simulink model "proyecto"  (R2021a)
settings: Solver=VariableStepAuto  StartTime=0.0  StopTime=10.0  RelTol=1e-3
model workspace (MAT data in the model file):
  Cts = Simulink.Parameter
  Cts.DataType = 'auto'
  Cts.Dimensions = [0 0]
  J_eq = Simulink.Parameter
  J_eq.DataType = 'auto'
  J_eq.Dimensions = [0 0]
  Jeq = Simulink.Parameter
  Jeq.DataType = 'auto'
  Jeq.Dimensions = [0 0]
  Ke = Simulink.Parameter
  Ke.DataType = 'auto'
  Ke.Dimensions = [0 0]
  Ksa = Simulink.Parameter
  Ksa.DataType = 'auto'
  Ksa.Dimensions = [0 0]
  Ksia = Simulink.Parameter
  Ksia.DataType = 'auto'
  Ksia.Dimensions = [0 0]
  Kt = Simulink.Parameter
  Kt.DataType = 'auto'
  Kt.Dimensions = [0 0]
  Ktheta = Simulink.Parameter
  Ktheta.DataType = 'auto'
  Ktheta.Dimensions = [0 0]
  Kw = Simulink.Parameter
  Kw.DataType = 'auto'
  Kw.Dimensions = [0 0]
  Ld = Simulink.Parameter
  Ld.DataType = 'auto'
  Ld.Dimensions = [0 0]
  LdP = Simulink.Parameter
  LdP.DataType = 'auto'
  LdP.Dimensions = [0 0]
  Lls = Simulink.Parameter
  Lls.DataType = 'auto'
  Lls.Dimensions = [0 0]
  Lq = Simulink.Parameter
  Lq.DataType = 'auto'
  Lq.Dimensions = [0 0]
  LqP = Simulink.Parameter
  LqP.DataType = 'auto'
  LqP.Dimensions = [0 0]
  Pp = Simulink.Parameter
  Pp.DataType = 'auto'
  Pp.Dimensions = [0 0]
  R0 = Simulink.Parameter
  R0.DataType = 'auto'
  R0.Dimensions = [0 0]
  R0P = Simulink.Parameter
  R0P.DataType = 'auto'
  R0P.Dimensions = [0 0]
  Rd = Simulink.Parameter
  Rd.DataType = 'auto'
  Rd.Dimensions = [0 0]
  RdP = Simulink.Parameter
  RdP.DataType = 'auto'
  RdP.Dimensions = [0 0]
  Rq = Simulink.Parameter
  Rq.DataType = 'auto'
  Rq.Dimensions = [0 0]
  RqP = Simulink.Parameter
  RqP.DataType = 'auto'
  RqP.Dimensions = [0 0]
  Rs = Simulink.Parameter
  Rs.DataType = 'auto'
  Rs.Dimensions = [0 0]
  RsP = Simulink.Parameter
  RsP.DataType = 'auto'
  RsP.Dimensions = [0 0]
  Rs_ref = Simulink.Parameter
  Rs_ref.DataType = 'auto'
  Rs_ref.Dimensions = [0 0]
  Rtsamb = Simulink.Parameter
  Rtsamb.DataType = 'auto'
  Rtsamb.Dimensions = [0 0]
  T_amb = Simulink.Parameter
  T_amb.DataType = 'auto'
  T_amb.Dimensions = [0 0]
  Ts_ref = Simulink.Parameter
  Ts_ref.DataType = 'auto'
  Ts_ref.Dimensions = [0 0]
  a_cu = Simulink.Parameter
  a_cu.DataType = 'auto'
  a_cu.Dimensions = [0 0]
  b_eq = Simulink.Parameter
  b_eq.DataType = 'auto'
  b_eq.Dimensions = [0 0]
  ba = Simulink.Parameter
  ba.DataType = 'auto'
  ba.Dimensions = [0 0]
  beqP = Simulink.Parameter
  beqP.DataType = 'auto'
  beqP.Dimensions = [0 0]
  lambda_m = Simulink.Parameter
  lambda_m.DataType = 'auto'
  lambda_m.Dimensions = [0 0]
  r = Simulink.Parameter
  r.DataType = 'auto'
  r.Dimensions = [0 0]
values from neighbouring files (symbols this model uses):
  a_cu = 3.9e-3    (= 0.0039)    [Datos.m]
  b_eq = 15.000e-6    (= 1.5e-05)    [Datos.m]
  ba = 0.0113    [Datos.m]
  Cts = 0.818    [Datos.m]
  Id_0 = 0    [Datos.m]
  J_eq = 5.6509e-6    (= 5.6509e-06)    [Datos.m]
  Ksa = 9.0414    [Datos.m]
  Ksia = 2893.2608    [Datos.m]
  Ktheta = 6397.34    [Datos.m]
  Kw = 10.2234e6    (= 10223400)    [Datos.m]
  lambda_m = 0.01546    [Datos.m]
  Ld = 6.6e-3    (= 0.0066)    [Datos.m]
  Lls = 0.8e-3    (= 0.0008)    [Datos.m]
  Lq = 5.8e-3    (= 0.0058)    [Datos.m]
  Pp = 3.01    [Datos.m]
  r = 314.3008    [Datos.m]
  Rs = 1.02    [Datos.m]
  Rs_ref = 1.02    [Datos.m]
  Rtsamb = 146.7    [Datos.m]
  T_0 = 40.0    (= 40)    [Datos.m]
  T_amb = 40    [Datos.m]
  Ts_ref = 40    [Datos.m]
undefined symbols (not defined in the file or in its folder): sigbuilder_block
(part 1 of 3)
settings Model: Creator=jpss8  LastModifiedBy=jpss8

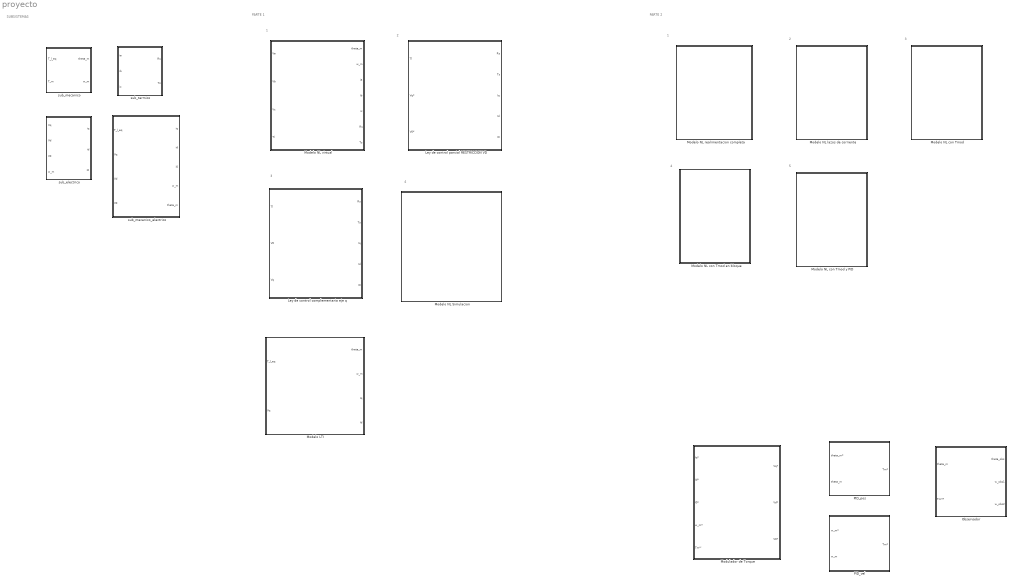
== system proyecto ==
  note: 1
  note: PARTE 2
  note: PARTE 1
  note: SUBSISTEMAS
  note: 2
  note: 3
  note: 4
  note: 5
  note: 1
  note: 2
  note: 3
  note: 4
  Ley de control complementaria eje q : Subsystem
  Ley de control parcial RESTRICCION VD : Subsystem
  Modelo LTI : Subsystem
  Modelo NL Simulacion : Subsystem
  Modelo NL con Tmod : Subsystem
  Modelo NL con Tmod en bloque : Subsystem
  Modelo NL con Tmod y PID : Subsystem
  Modelo NL lazos de corriente : Subsystem
  Modelo NL realimentacion completa : Subsystem
  Modelo NL virtual : Subsystem
  Modulador de Torque : Subsystem
  Observador : Subsystem
  PID_pos : Subsystem
  PID_vel : Subsystem
  sub_electrico : Subsystem
  sub_mecanico : Subsystem
  sub_mecanico_electrico : Subsystem
  sub_termico : Subsystem

== system proyecto/Ley de control complementaria eje q ==
  note: CONTROLADOR (Ley complementaria eje q)
  note: SISTEMA FÍSICO
  Tl : Inport
  V0 : Inport  Port=2
  Vq : Inport  Port=3
  Constant : Constant  Value=lambda_m
  Gain : Gain  Gain=Pp
  Gain1 : Gain  Gain=1/r
  Gain2 : Gain  Gain=Pp
  Gain3 : Gain  Gain=-Lq
  Gain4 : Gain  Gain=Ld
  Gain8 : Gain  Gain=Pp
  Modulador de Tensión : Subsystem
  Product : Product
  Product1 : Product
  Sensor de Corriente : Subsystem
  Sensor de posición : Gain
  Sensor de velocidad : Gain
  Sum : Sum  Inputs=|++
  Sum1 : Sum  Inputs=|++
  inverse_park_transform : MATLAB Function  TreatAsAtomicUnit=on
  inverse_park_transform1 : MATLAB Function  TreatAsAtomicUnit=on
  park_transform : MATLAB Function  TreatAsAtomicUnit=on
  park_transform1 : MATLAB Function  TreatAsAtomicUnit=on
  sub_mecanico_electrico : Subsystem
  sub_termico : Subsystem
  Rs : Outport
  Ts : Outport  Port=2
  Iq : Outport  Port=3
  Id : Outport  Port=4
  I0 : Outport  Port=5
  wires:
  Gain/1 -> inverse_park_transform/4(theta_r), park_transform/4(theta_r)
  Tl/1 -> Gain1/1
  Gain1/1 -> sub_mecanico_electrico/4(V0)
  sub_mecanico_electrico/1(iq) -> inverse_park_transform/1(fq)
  park_transform/1(fq) -> sub_mecanico_electrico/1(T_l_eq)
  park_transform/2(fd) -> sub_mecanico_electrico/2(Vq)
  sub_mecanico_electrico/2(id) -> inverse_park_transform/2(fd)
  sub_mecanico_electrico/3(i0) -> inverse_park_transform/3(f0)
  sub_mecanico_electrico/5(theta_m) -> Sensor de posición/1, Gain/1
  sub_termico/1(Rs) -> Rs/1
  sub_termico/2(Ts) -> Ts/1
  sub_mecanico_electrico/4(w_m) -> Sensor de velocidad/1
  park_transform/3(f0) -> sub_mecanico_electrico/3(Vd)
  Gain8/1 -> park_transform1/4(theta_r), inverse_park_transform1/4(theta_r)  "theta_r*"
  Modulador de Tensión/1(Out1) -> park_transform/1(fa)  "Va"
  Modulador de Tensión/2(Out2) -> park_transform/2(fb)  "Vb"
  Modulador de Tensión/3(Out3) -> park_transform/3(fc)  "Vc"
  Sensor de Corriente/1(Out1) -> park_transform1/1(fa), sub_termico/1(ia)
  Sensor de Corriente/3(Out3) -> park_transform1/3(fc), sub_termico/3(ic)
  Sensor de Corriente/2(Out2) -> sub_termico/2(ib), park_transform1/2(fb)
  inverse_park_transform/1(fa) -> Sensor de Corriente/1(In1)
  inverse_park_transform/2(fb) -> Sensor de Corriente/2(In2)
  inverse_park_transform/3(fc) -> Sensor de Corriente/3(In3)
  park_transform1/1(fq) -> Gain3/1, Iq/1  "Iq*"
  park_transform1/2(fd) -> Gain4/1, Id/1  "Id*"
  park_transform1/3(f0) -> I0/1  "I0*"
  Product/1 -> inverse_park_transform1/2(fd)  "Vd*"
  V0/1 -> inverse_park_transform1/3(f0)
  inverse_park_transform1/2(fb) -> Modulador de Tensión/2(fb)  "Vb*"
  inverse_park_transform1/3(fc) -> Modulador de Tensión/3(fc)  "Vc*"
  inverse_park_transform1/1(fa) -> Modulador de Tensión/1(fa)  "Va*"
  Sensor de posición/1 -> Gain8/1  "theta_m*"
  Sensor de velocidad/1 -> Gain2/1  "w_m*"
  Gain2/1 -> Product1/1, Product/1
  Gain3/1 -> Product/2
  Gain4/1 -> Sum/1
  Sum/1 -> Product1/2  "lambda_m + Ld*Id"
  Constant/1 -> Sum/2
  Product1/1 -> Sum1/2
  Sum1/1 -> inverse_park_transform1/1(fq)  "Vq*"
  Vq/1 -> Sum1/1

== system proyecto/Ley de control parcial RESTRICCION VD ==
  note: CONTROLADOR (Restricción Vd)
  note: SISTEMA FÍSICO
  Tl : Inport
  Vq* : Inport  Port=2
  V0* : Inport  Port=3
  Gain : Gain  Gain=Pp
  Gain1 : Gain  Gain=1/r
  Gain2 : Gain  Gain=Pp
  Gain3 : Gain  Gain=-Lq
  Gain8 : Gain  Gain=Pp
  Modulador de Tensión : Subsystem
  Product : Product
  Sensor de Corriente : Subsystem
  Sensor de posición : Gain
  Sensor de velocidad : Gain
  inverse_park_transform : MATLAB Function  TreatAsAtomicUnit=on
  inverse_park_transform1 : MATLAB Function  TreatAsAtomicUnit=on
  park_transform : MATLAB Function  TreatAsAtomicUnit=on
  park_transform1 : MATLAB Function  TreatAsAtomicUnit=on
  sub_mecanico_electrico : Subsystem
  sub_termico : Subsystem
  Rs : Outport
  Ts : Outport  Port=2
  Iq : Outport  Port=3
  Id : Outport  Port=4
  I0 : Outport  Port=5
  wires:
  Gain/1 -> inverse_park_transform/4(theta_r), park_transform/4(theta_r)
  Tl/1 -> Gain1/1
  Gain1/1 -> sub_mecanico_electrico/4(V0)
  sub_mecanico_electrico/1(iq) -> inverse_park_transform/1(fq)
  park_transform/1(fq) -> sub_mecanico_electrico/1(T_l_eq)
  park_transform/2(fd) -> sub_mecanico_electrico/2(Vq)
  sub_mecanico_electrico/2(id) -> inverse_park_transform/2(fd)
  sub_mecanico_electrico/3(i0) -> inverse_park_transform/3(f0)
  sub_mecanico_electrico/5(theta_m) -> Sensor de posición/1, Gain/1
  sub_termico/1(Rs) -> Rs/1
  sub_termico/2(Ts) -> Ts/1
  sub_mecanico_electrico/4(w_m) -> Sensor de velocidad/1
  park_transform/3(f0) -> sub_mecanico_electrico/3(Vd)
  Gain8/1 -> park_transform1/4(theta_r), inverse_park_transform1/4(theta_r)  "theta_r*"
  Modulador de Tensión/1(Out1) -> park_transform/1(fa)  "Va"
  Modulador de Tensión/2(Out2) -> park_transform/2(fb)  "Vb"
  Modulador de Tensión/3(Out3) -> park_transform/3(fc)  "Vc"
  Sensor de Corriente/1(Out1) -> park_transform1/1(fa), sub_termico/1(ia)
  Sensor de Corriente/3(Out3) -> sub_termico/3(ic), park_transform1/3(fc)
  Sensor de Corriente/2(Out2) -> sub_termico/2(ib), park_transform1/2(fb)
  inverse_park_transform/1(fa) -> Sensor de Corriente/1(In1)
  inverse_park_transform/2(fb) -> Sensor de Corriente/2(In2)
  inverse_park_transform/3(fc) -> Sensor de Corriente/3(In3)
  park_transform1/1(fq) -> Gain3/1, Iq/1  "Iq*"
  park_transform1/2(fd) -> Id/1
  park_transform1/3(f0) -> I0/1
  Vq*/1 -> inverse_park_transform1/1(fq)
  Product/1 -> inverse_park_transform1/2(fd)  "Vd*"
  V0*/1 -> inverse_park_transform1/3(f0)
  inverse_park_transform1/2(fb) -> Modulador de Tensión/2(fb)  "Vb*"
  inverse_park_transform1/3(fc) -> Modulador de Tensión/3(fc)  "Vc*"
  inverse_park_transform1/1(fa) -> Modulador de Tensión/1(fa)  "Va*"
  Sensor de posición/1 -> Gain8/1  "theta_m*"
  Sensor de velocidad/1 -> Gain2/1  "w_m*"
  Gain2/1 -> Product/1
  Gain3/1 -> Product/2

== system proyecto/Modelo LTI ==
  T_l_eq : Inport
  Vq : Inport  Port=2
  Constant1 : Constant  Value=0
  Gain : Gain  Gain=3/2*Pp*lambda_m
  Gain1 : Gain  Gain=Pp*lambda_m
  Gain12 : Gain  Gain=Rs
  Gain13 : Gain  Gain=1/Ld
  Gain2 : Gain  Gain=Rs
  Gain3 : Gain  Gain=1/Lq
  Gain4 : Gain  Gain=1/J_eq
  Gain5 : Gain  Gain=b_eq
  Integrator{,1..3} (4 alike) : Integrator
  Sum : Sum  Inputs=-+-
  Sum1 : Sum  Inputs=+--
  Sum5 : Sum  Inputs=|+-
  theta_m : Outport
  w_m : Outport  Port=2
  Iq : Outport  Port=3
  Id : Outport  Port=4
  wires:
  Integrator1/1 -> theta_m/1
  Gain4/1 -> Integrator/1
  T_l_eq/1 -> Sum/1
  Sum/1 -> Gain4/1
  Integrator/1 -> Integrator1/1, Gain1/1, Gain5/1, w_m/1
  Gain5/1 -> Sum/3
  Gain/1 -> Sum/2
  Vq/1 -> Sum1/1
  Gain1/1 -> Sum1/2
  Gain2/1 -> Sum1/3
  Sum1/1 -> Gain3/1
  Gain3/1 -> Integrator2/1
  Integrator2/1 -> Iq/1, Gain2/1, Gain/1  "Iq"
  Integrator3/1 -> Id/1, Gain12/1  "Id"
  Sum5/1 -> Gain13/1
  Gain13/1 -> Integrator3/1
  Constant1/1 -> Sum5/1
  Gain12/1 -> Sum5/2

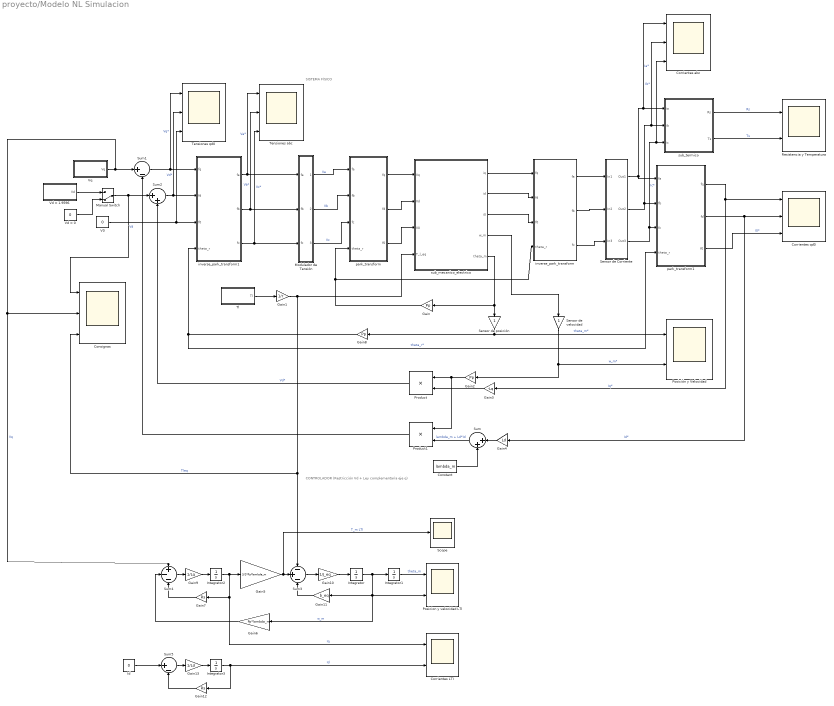
== system proyecto/Modelo NL Simulacion ==
  note: SISTEMA FÍSICO
  note: CONTROLADOR (Restricción Vd + Ley complementaria eje q)
  Consignas : Scope  NumInputPorts=3
  Constant : Constant  Value=lambda_m
  Corrientes LTI : Scope  NumInputPorts=2
  Corrientes abc : Scope  NumInputPorts=3
  Corrientes qd0 : Scope  NumInputPorts=3
  Gain : Gain  Gain=Pp
  Gain1 : Gain  Gain=1/r
  Gain10 : Gain  Gain=1/J_eq
  Gain11 : Gain  Gain=b_eq
  Gain12 : Gain  Gain=Rs
  Gain13 : Gain  Gain=1/Ld
  Gain2 : Gain  Gain=Pp
  Gain3 : Gain  Gain=-Lq
  Gain4 : Gain  Gain=Ld
  Gain5 : Gain  Gain=3/2*Pp*lambda_m
  Gain6 : Gain  Gain=Pp*lambda_m
  Gain7 : Gain  Gain=Rs
  Gain8 : Gain  Gain=Pp
  Gain9 : Gain  Gain=1/Lq
  Id : Constant  Value=0
  Integrator : Integrator
  Integrator1 : Integrator
  Integrator2 : Integrator
  Integrator3 : Integrator  InitialCondition=Id_0
  Manual Switch : ManualSwitch  CurrentSetting=0
  Modulador de Tensión : Subsystem
  Posicion y velocidad LTI : Scope  NumInputPorts=2
  Posición y Velocidad : Scope  NumInputPorts=2
  Product : Product
  Product1 : Product
  Resistencia y Temperatura : Scope  NumInputPorts=2
  Scope : Scope
  Sensor de Corriente : Subsystem
  Sensor de posición : Gain
  Sensor de velocidad : Gain
  Sum : Sum  Inputs=|++
  Sum1 : Sum  Inputs=|+-
  Sum2 : Sum  Inputs=|++
  Sum3 : Sum  Inputs=-+-
  Sum4 : Sum  Inputs=+--
  Sum5 : Sum  Inputs=|+-
  Tensiones abc : Scope  NumInputPorts=3
  Tensiones qd0 : Scope  NumInputPorts=3
  Tl : Subsystem  Tag=STV Subsys  LoadFcn=sigbuilder_block('load');  StartFcn=sigbuilder_block('start');  StopFcn=sigbuilder_block('stop');  ClipboardFcn=sigbuilder_block('clipboard');  mask(Sigbuilder block){tuvar=[0:10]}
      mask help: Simulink:masks:SigbuilderBlock_MD
      mask init:
      | if ~strcmp(get_param(bdroot(gcbh),'SimulationStatus'),'stopped') tuvar = sigbuilder_block('maskInit'); end
      settings: CopyFcn=sigbuilder_block('copy');  DeleteFcn=sigbuilder_block('delete');  ModelCloseFcn=sigbuilder_block('modelClose');  PreSaveFcn=sigbuilder_block('preSave');  PauseFcn=sigbuilder_block('pause');  ContinueFcn=sigbuilder_block('continue');  NameChangeFcn=sigbuilder_block('namechange');  OpenFcn=sigbuilder_block('open',[5.5 30 1269 678 ]);  CloseFcn=sigbuilder_block('close');
      mask Display: plot(0, 0, 100, 100,[2, 2, 32, 32, 2], [68, 8, 8, 68, 68],[32, 2], [38, 38], [32, 19, 2],[53, 60, 44], [32, 17, 17, 2],[16, 16, 31, 31]);txt = getActiveGroup(gcbh);text(2, 100, txt,'verticalAlignment', 'top');
  V0 : Constant  Value=0
  Vd = 0 : Constant  Value=0
  Vd = 1.9596 : Subsystem  Tag=STV Subsys  LoadFcn=sigbuilder_block('load');  StartFcn=sigbuilder_block('start');  StopFcn=sigbuilder_block('stop');  ClipboardFcn=sigbuilder_block('clipboard');  mask(Sigbuilder block){tuvar=[0:10]}
      mask help: Simulink:masks:SigbuilderBlock_MD
      mask init:
      | if ~strcmp(get_param(bdroot(gcbh),'SimulationStatus'),'stopped') tuvar = sigbuilder_block('maskInit'); end
      settings: CopyFcn=sigbuilder_block('copy');  DeleteFcn=sigbuilder_block('delete');  ModelCloseFcn=sigbuilder_block('modelClose');  PreSaveFcn=sigbuilder_block('preSave');  PauseFcn=sigbuilder_block('pause');  ContinueFcn=sigbuilder_block('continue');  NameChangeFcn=sigbuilder_block('namechange');  OpenFcn=sigbuilder_block('open',[5.5 30 1269 678 ]);  CloseFcn=sigbuilder_block('close');
      mask Display: plot(0, 0, 100, 100,[2, 2, 32, 32, 2], [68, 8, 8, 68, 68],[32, 2], [38, 38], [32, 19, 2],[53, 60, 44], [32, 17, 17, 2],[16, 16, 31, 31]);txt = getActiveGroup(gcbh);text(2, 100, txt,'verticalAlignment', 'top');
  Vq : Subsystem  Tag=STV Subsys  LoadFcn=sigbuilder_block('load');  StartFcn=sigbuilder_block('start');  StopFcn=sigbuilder_block('stop');  ClipboardFcn=sigbuilder_block('clipboard');  mask(Sigbuilder block){tuvar=[0:10]}
      mask help: Simulink:masks:SigbuilderBlock_MD
      mask init:
      | if ~strcmp(get_param(bdroot(gcbh),'SimulationStatus'),'stopped') tuvar = sigbuilder_block('maskInit'); end
      settings: CopyFcn=sigbuilder_block('copy');  DeleteFcn=sigbuilder_block('delete');  ModelCloseFcn=sigbuilder_block('modelClose');  PreSaveFcn=sigbuilder_block('preSave');  PauseFcn=sigbuilder_block('pause');  ContinueFcn=sigbuilder_block('continue');  NameChangeFcn=sigbuilder_block('namechange');  OpenFcn=sigbuilder_block('open',[5.5 30 1269 678 ]);  CloseFcn=sigbuilder_block('close');
      mask Display: plot(0, 0, 100, 100,[2, 2, 32, 32, 2], [68, 8, 8, 68, 68],[32, 2], [38, 38], [32, 19, 2],[53, 60, 44], [32, 17, 17, 2],[16, 16, 31, 31]);txt = getActiveGroup(gcbh);text(2, 100, txt,'verticalAlignment', 'top');
  inverse_park_transform : MATLAB Function  TreatAsAtomicUnit=on
  inverse_park_transform1 : MATLAB Function  TreatAsAtomicUnit=on
  park_transform : MATLAB Function  TreatAsAtomicUnit=on
  park_transform1 : MATLAB Function  TreatAsAtomicUnit=on
  sub_mecanico_electrico : Subsystem
  sub_termico : Subsystem
  wires:
  park_transform1/3(f0) -> Corrientes qd0/3  "I0*"
  Product1/1 -> Sum1/2
  inverse_park_transform/2(fb) -> Sensor de Corriente/2(In2)
  Integrator1/1 -> Posicion y velocidad LTI/1  "theta_m"
  sub_termico/1(Rs) -> Resistencia y Temperatura/1  "Rs"
  Gain6/1 -> Sum4/2
  Gain5/1 -> Scope/1, Sum3/2  "T_m LTI"
  Sensor de Corriente/1(Out1) -> park_transform1/1(fa), Corrientes abc/1, sub_termico/1(ia)  "Ia*"
  Gain13/1 -> Integrator3/1
  sub_mecanico_electrico/1(iq) -> inverse_park_transform/1(fq)
  Gain7/1 -> Sum4/3
  Modulador de Tensión/1(Out1) -> park_transform/1(fa)  "Va"
  park_transform/1(fq) -> sub_mecanico_electrico/1(Vq)
  Id/1 -> Sum5/1
  Sum5/1 -> Gain13/1
  Gain12/1 -> Sum5/2
  park_transform1/1(fq) -> Gain3/1, Corrientes qd0/1  "Iq*"
  Sum2/1 -> Tensiones qd0/2, inverse_park_transform1/2(fd)  "Vd*"
  Gain9/1 -> Integrator2/1
  Gain11/1 -> Sum3/3
  park_transform1/2(fd) -> Gain4/1, Corrientes qd0/2  "Id*"
  Gain10/1 -> Integrator/1
  Sum4/1 -> Gain9/1
  Gain8/1 -> park_transform1/4(theta_r), inverse_park_transform1/4(theta_r)  "theta_r*"
  Sum3/1 -> Gain10/1
  Integrator2/1 -> Gain7/1, Corrientes LTI/1, Gain5/1  "Iq"
  Integrator/1 -> Gain6/1, Posicion y velocidad LTI/2, Gain11/1, Integrator1/1  "w_m"
  Vd = 0/1 -> Manual Switch/2
  Modulador de Tensión/3(Out3) -> park_transform/3(fc)  "Vc"
  park_transform/3(f0) -> sub_mecanico_electrico/3(V0)
  Sensor de velocidad/1 -> Gain2/1, Posición y Velocidad/2  "w_m*"
  Vd = 1.9596/1(Vd) -> Manual Switch/1
  park_transform/2(fd) -> sub_mecanico_electrico/2(Vd)
  Sensor de Corriente/2(Out2) -> park_transform1/2(fb), Corrientes abc/2, sub_termico/2(ib)  "Ib*"
  inverse_park_transform/3(fc) -> Sensor de Corriente/3(In3)
  Manual Switch/1 -> Consignas/1, Sum2/1  "Vd"
  Sensor de Corriente/3(Out3) -> park_transform1/3(fc), Corrientes abc/3, sub_termico/3(ic)  "Ic*"
  inverse_park_transform1/1(fa) -> Tensiones abc/1, Modulador de Tensión/1(fa)  "Va*"
  Tl/1(Tl) -> Gain1/1
  sub_mecanico_electrico/4(w_m) -> Sensor de velocidad/1
  Gain3/1 -> Product/2
  inverse_park_transform/1(fa) -> Sensor de Corriente/1(In1)
  Modulador de Tensión/2(Out2) -> park_transform/2(fb)  "Vb"
  Gain/1 -> inverse_park_transform/4(theta_r), park_transform/4(theta_r)
  Sum/1 -> Product1/2  "lambda_m + Ld*Id"
  Product/1 -> Sum2/2  "Vd*"
  Constant/1 -> Sum/2
  Sum1/1 -> Tensiones qd0/1, inverse_park_transform1/1(fq)  "Vq*"
  Integrator3/1 -> Gain12/1, Corrientes LTI/2  "Id"
  Gain4/1 -> Sum/1
  sub_mecanico_electrico/5(theta_m) -> Sensor de posición/1, Gain/1
  V0/1 -> inverse_park_transform1/3(f0), Tensiones qd0/3
  sub_mecanico_electrico/3(i0) -> inverse_park_transform/3(f0)
  Gain1/1 -> Consignas/3, Sum3/1, sub_mecanico_electrico/4(T_l_eq)  "Tleq"
  sub_termico/2(Ts) -> Resistencia y Temperatura/2  "Ts"
  Gain2/1 -> Product1/1, Product/1
  inverse_park_transform1/2(fb) -> Modulador de Tensión/2(fb), Tensiones abc/2  "Vb*"
  Vq/1(Vq) -> Sum1/1, Consignas/2, Sum4/1  "Vq"
  sub_mecanico_electrico/2(id) -> inverse_park_transform/2(fd)
  inverse_park_transform1/3(fc) -> Modulador de Tensión/3(fc), Tensiones abc/3  "Vc*"
  Sensor de posición/1 -> Gain8/1, Posición y Velocidad/1  "theta_m*"

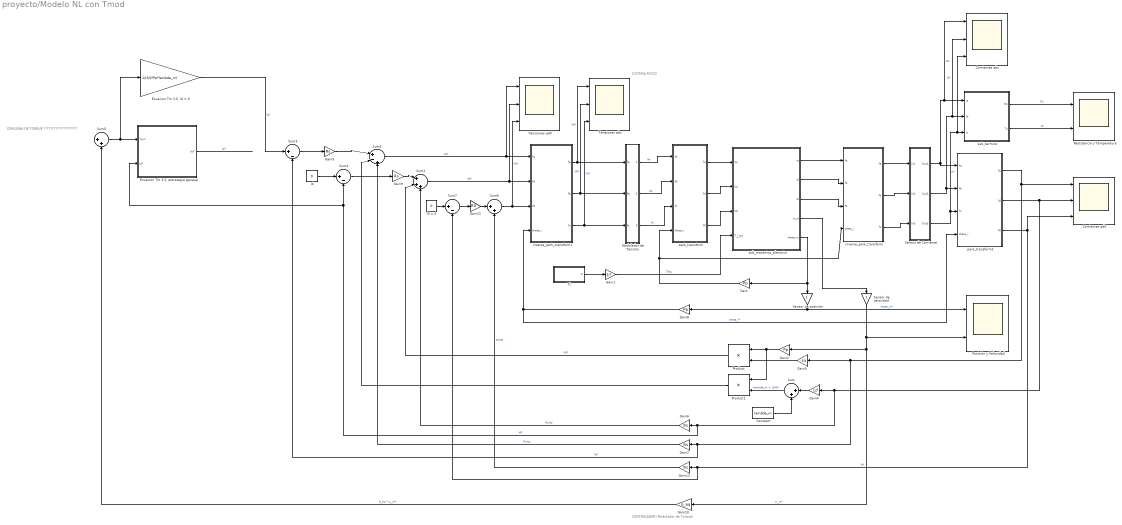
== system proyecto/Modelo NL con Tmod ==
  note: CONSIGNA DE TORQUE ????????????????????
  note: CONTROLADOR (Modulador de Torque)
  note: SISTEMA FÍSICO
  Constant : Constant  Value=lambda_m
  Corrientes abc : Scope  NumInputPorts=3
  Corrientes qd0 : Scope  NumInputPorts=3
  "Ecuacion Tm 3.5, Id = 0" : Gain  Gain=1/(3/2*Pp*lambda_m)
  "Ecuacion Tm 3.5, estrategia general" : Subsystem
  Gain : Gain  Gain=Pp
  Gain1 : Gain  Gain=1/r
  Gain10 : Gain  Gain=b_eq
  Gain11 : Gain  Gain=R0
  Gain{5..7,9,12} (5 alike) : Gain  Gain=Rs
  Gain2 : Gain  Gain=Pp
  Gain3 : Gain  Gain=-Lq
  Gain4 : Gain  Gain=Ld
  Gain8 : Gain  Gain=Pp
  I0 = 0 : Constant  Value=0
  Id : Constant  Value=0
  Modulador de Tensión : Subsystem
  Posición y Velocidad : Scope  NumInputPorts=2
  Product : Product
  Product1 : Product
  Resistencia y Temperatura : Scope  NumInputPorts=2
  Sensor de Corriente : Subsystem
  Sensor de posición : Gain
  Sensor de velocidad : Gain
  Sum : Sum  Inputs=|++
  Sum1 : Sum  Inputs=|+-+
  Sum2 : Sum  Inputs=|+++
  Sum3 : Sum  Inputs=|+-
  Sum4 : Sum  Inputs=|+-
  Sum5 : Sum  Inputs=|++
  Sum6 : Sum  Inputs=|++
  Sum7 : Sum  Inputs=|+-
  Tensiones abc : Scope  NumInputPorts=3
  Tensiones qd0 : Scope  NumInputPorts=3
  Tl : Subsystem  Tag=STV Subsys  LoadFcn=sigbuilder_block('load');  StartFcn=sigbuilder_block('start');  StopFcn=sigbuilder_block('stop');  ClipboardFcn=sigbuilder_block('clipboard');  mask(Sigbuilder block){tuvar=[0:10]}
      mask help: Simulink:masks:SigbuilderBlock_MD
      mask init:
      | if ~strcmp(get_param(bdroot(gcbh),'SimulationStatus'),'stopped') tuvar = sigbuilder_block('maskInit'); end
      settings: CopyFcn=sigbuilder_block('copy');  DeleteFcn=sigbuilder_block('delete');  ModelCloseFcn=sigbuilder_block('modelClose');  PreSaveFcn=sigbuilder_block('preSave');  PauseFcn=sigbuilder_block('pause');  ContinueFcn=sigbuilder_block('continue');  NameChangeFcn=sigbuilder_block('namechange');  OpenFcn=sigbuilder_block('open',[5.5 30 1269 678 ]);  CloseFcn=sigbuilder_block('close');
      mask Display: plot(0, 0, 100, 100,[2, 2, 32, 32, 2], [68, 8, 8, 68, 68],[32, 2], [38, 38], [32, 19, 2],[53, 60, 44], [32, 17, 17, 2],[16, 16, 31, 31]);txt = getActiveGroup(gcbh);text(2, 100, txt,'verticalAlignment', 'top');
  inverse_park_transform : MATLAB Function  TreatAsAtomicUnit=on
  inverse_park_transform1 : MATLAB Function  TreatAsAtomicUnit=on
  park_transform : MATLAB Function  TreatAsAtomicUnit=on
  park_transform1 : MATLAB Function  TreatAsAtomicUnit=on
  sub_mecanico_electrico : Subsystem
  sub_termico : Subsystem
  wires:
  Sum4/1 -> Gain9/1
  Tl/1(Tl) -> Gain1/1
  inverse_park_transform/3(fc) -> Sensor de Corriente/3(In3)
  Sensor de Corriente/3(Out3) -> park_transform1/3(fc), Corrientes abc/3, sub_termico/3(ic)  "Ic*"
  Gain3/1 -> Product/2
  Product1/1 -> Sum1/2
  inverse_park_transform/2(fb) -> Sensor de Corriente/2(In2)
  sub_termico/1(Rs) -> Resistencia y Temperatura/1  "Rs"
  Modulador de Tensión/1(Out1) -> park_transform/1(fa)  "Va"
  Sensor de Corriente/1(Out1) -> park_transform1/1(fa), Corrientes abc/1, sub_termico/1(ia)  "Ia*"
  park_transform/1(fq) -> sub_mecanico_electrico/1(Vq)
  sub_mecanico_electrico/1(iq) -> inverse_park_transform/1(fq)
  Sum1/1 -> Tensiones qd0/1, inverse_park_transform1/1(fq)  "Vq*"
  park_transform1/1(fq) -> Sum3/2, Gain7/1, Gain3/1, Corrientes qd0/1  "Iq*"
  park_transform/3(f0) -> sub_mecanico_electrico/3(V0)
  Sum6/1 -> inverse_park_transform1/3(f0), Tensiones qd0/3  "V0*"
  park_transform/2(fd) -> sub_mecanico_electrico/2(Vd)
  Gain8/1 -> park_transform1/4(theta_r), inverse_park_transform1/4(theta_r)  "theta_r*"
  park_transform1/2(fd) -> Sum4/2, "Ecuacion Tm 3.5, estrategia general"/2(Id*), Gain6/1, Gain4/1, Corrientes qd0/2  "Id*"
  inverse_park_transform/1(fa) -> Sensor de Corriente/1(In1)
  Gain4/1 -> Sum/1
  Gain/1 -> inverse_park_transform/4(theta_r), park_transform/4(theta_r)
  sub_mecanico_electrico/5(theta_m) -> Sensor de posición/1, Gain/1
  Constant/1 -> Sum/2
  sub_mecanico_electrico/3(i0) -> inverse_park_transform/3(f0)
  Gain1/1 -> sub_mecanico_electrico/4(T_l_eq)  "Tleq"
  Gain2/1 -> Product1/1, Product/1
  Sensor de velocidad/1 -> Gain2/1, Gain10/1, Posición y Velocidad/2  "w_m*"
  Sum/1 -> Product1/2  "lambda_m + Ld*Id"
  Modulador de Tensión/2(Out2) -> park_transform/2(fb)  "Vb"
  inverse_park_transform1/2(fb) -> Modulador de Tensión/2(fb), Tensiones abc/2  "Vb*"
  inverse_park_transform1/3(fc) -> Modulador de Tensión/3(fc), Tensiones abc/3  "Vc*"
  inverse_park_transform1/1(fa) -> Tensiones abc/1, Modulador de Tensión/1(fa)  "Va*"
  Sensor de posición/1 -> Gain8/1, Posición y Velocidad/1  "theta_m*"
  sub_mecanico_electrico/2(id) -> inverse_park_transform/2(fd)
  Modulador de Tensión/3(Out3) -> park_transform/3(fc)  "Vc"
  Gain6/1 -> Sum2/3  "Rs*Id"
  Sum2/1 -> Tensiones qd0/2, inverse_park_transform1/2(fd)  "Vd*"
  sub_mecanico_electrico/4(w_m) -> Sensor de velocidad/1
  Product/1 -> Sum2/2  "Vd*"
  Sensor de Corriente/2(Out2) -> park_transform1/2(fb), Corrientes abc/2, sub_termico/2(ib)  "Ib*"
  sub_termico/2(Ts) -> Resistencia y Temperatura/2  "Ts"
  Gain7/1 -> Sum1/3  "Rs*Iq"
  Sum3/1 -> Gain5/1
  Gain5/1 -> Sum1/1
  Gain9/1 -> Sum2/1
  Id/1 -> Sum4/1
  "Ecuacion Tm 3.5, estrategia general"/1(Iq*') -> ?  "Iq*'"
  Sum5/1 -> "Ecuacion Tm 3.5, Id = 0"/1, "Ecuacion Tm 3.5, estrategia general"/1(Tm*')
  ? -> Sum5/1
  Gain10/1 -> Sum5/2  "b_eq * w_m*"
  "Ecuacion Tm 3.5, Id = 0"/1 -> Sum3/1  "Iq*"
  Sum7/1 -> Gain11/1
  park_transform1/3(f0) -> Gain12/1, Sum7/2, Corrientes qd0/3  "I0*"
  I0 = 0/1 -> Sum7/1
  Gain11/1 -> Sum6/1
  Gain12/1 -> Sum6/2  "Rs*I0"

== system proyecto/Modelo NL con Tmod en bloque ==
  note: CONTROLADOR CON TMOD
  note: CONSIGNA DE TORQUE
  note: SISTEMA FÍSICO
  Corrientes abc : Scope  NumInputPorts=3
  Corrientes qd0 : Scope  NumInputPorts=3
  Gain : Gain  Gain=Pp
  Gain1 : Gain  Gain=1/r
  Gain8 : Gain  Gain=Pp
  Modulador de Tensión : Subsystem
  Modulador de Torque : Subsystem
  Posición y Velocidad : Scope  NumInputPorts=2
  Resistencia y Temperatura : Scope  NumInputPorts=2
  Sensor de Corriente : Subsystem
  Sensor de posición : Gain
  Sensor de velocidad : Gain
  Tensiones abc : Scope  NumInputPorts=3
  Tensiones qd0 : Scope  NumInputPorts=3
  Tl : Subsystem  Tag=STV Subsys  LoadFcn=sigbuilder_block('load');  StartFcn=sigbuilder_block('start');  StopFcn=sigbuilder_block('stop');  ClipboardFcn=sigbuilder_block('clipboard');  mask(Sigbuilder block){tuvar=[0:10]}
      mask help: Simulink:masks:SigbuilderBlock_MD
      mask init:
      | if ~strcmp(get_param(bdroot(gcbh),'SimulationStatus'),'stopped') tuvar = sigbuilder_block('maskInit'); end
      settings: CopyFcn=sigbuilder_block('copy');  DeleteFcn=sigbuilder_block('delete');  ModelCloseFcn=sigbuilder_block('modelClose');  PreSaveFcn=sigbuilder_block('preSave');  PauseFcn=sigbuilder_block('pause');  ContinueFcn=sigbuilder_block('continue');  NameChangeFcn=sigbuilder_block('namechange');  OpenFcn=sigbuilder_block('open',[5.5 30 1269 678 ]);  CloseFcn=sigbuilder_block('close');
      mask Display: plot(0, 0, 100, 100,[2, 2, 32, 32, 2], [68, 8, 8, 68, 68],[32, 2], [38, 38], [32, 19, 2],[53, 60, 44], [32, 17, 17, 2],[16, 16, 31, 31]);txt = getActiveGroup(gcbh);text(2, 100, txt,'verticalAlignment', 'top');
  inverse_park_transform : MATLAB Function  TreatAsAtomicUnit=on
  inverse_park_transform1 : MATLAB Function  TreatAsAtomicUnit=on
  park_transform : MATLAB Function  TreatAsAtomicUnit=on
  park_transform1 : MATLAB Function  TreatAsAtomicUnit=on
  sub_mecanico_electrico : Subsystem
  sub_termico : Subsystem
  wires:
  Tl/1(Tl) -> Gain1/1
  inverse_park_transform/3(fc) -> Sensor de Corriente/3(In3)
  Sensor de Corriente/3(Out3) -> park_transform1/3(fc), Corrientes abc/3, sub_termico/3(ic)  "Ic*"
  inverse_park_transform/2(fb) -> Sensor de Corriente/2(In2)
  sub_termico/1(Rs) -> Resistencia y Temperatura/1  "Rs"
  Modulador de Tensión/1(Out1) -> park_transform/1(fa)  "Va"
  Sensor de Corriente/1(Out1) -> park_transform1/1(fa), Corrientes abc/1, sub_termico/1(ia)  "Ia*"
  park_transform/1(fq) -> sub_mecanico_electrico/1(Vq)
  sub_mecanico_electrico/1(iq) -> inverse_park_transform/1(fq)
  park_transform1/1(fq) -> Modulador de Torque/2(Iq*), Corrientes qd0/1  "Iq*"
  park_transform/3(f0) -> sub_mecanico_electrico/3(V0)
  park_transform/2(fd) -> sub_mecanico_electrico/2(Vd)
  Gain8/1 -> park_transform1/4(theta_r), inverse_park_transform1/4(theta_r)  "theta_r*"
  park_transform1/2(fd) -> Modulador de Torque/3(Id*), Corrientes qd0/2  "Id*"
  inverse_park_transform/1(fa) -> Sensor de Corriente/1(In1)
  Gain/1 -> inverse_park_transform/4(theta_r), park_transform/4(theta_r)
  sub_mecanico_electrico/5(theta_m) -> Sensor de posición/1, Gain/1
  sub_mecanico_electrico/3(i0) -> inverse_park_transform/3(f0)
  Gain1/1 -> sub_mecanico_electrico/4(T_l_eq)  "Tleq"
  Sensor de velocidad/1 -> Modulador de Torque/5(w_m*), Posición y Velocidad/2  "w_m*"
  Modulador de Tensión/2(Out2) -> park_transform/2(fb)  "Vb"
  inverse_park_transform1/2(fb) -> Modulador de Tensión/2(fb), Tensiones abc/2  "Vb*"
  inverse_park_transform1/3(fc) -> Modulador de Tensión/3(fc), Tensiones abc/3  "Vc*"
  inverse_park_transform1/1(fa) -> Tensiones abc/1, Modulador de Tensión/1(fa)  "Va*"
  Sensor de posición/1 -> Gain8/1, Posición y Velocidad/1  "theta_m*"
  sub_mecanico_electrico/2(id) -> inverse_park_transform/2(fd)
  Modulador de Tensión/3(Out3) -> park_transform/3(fc)  "Vc"
  sub_mecanico_electrico/4(w_m) -> Sensor de velocidad/1
  Sensor de Corriente/2(Out2) -> park_transform1/2(fb), Corrientes abc/2, sub_termico/2(ib)  "Ib*"
  sub_termico/2(Ts) -> Resistencia y Temperatura/2  "Ts"
  park_transform1/3(f0) -> Modulador de Torque/4(I0*), Corrientes qd0/3  "I0*"
  Modulador de Torque/1(Vq*) -> Tensiones qd0/1, inverse_park_transform1/1(fq)  "Vq*"
  Modulador de Torque/2(Vd*) -> Tensiones qd0/2, inverse_park_transform1/2(fd)  "Vd*"
  Modulador de Torque/3(V0*) -> inverse_park_transform1/3(f0), Tensiones qd0/3  "V0*"
  ? -> Modulador de Torque/1(Tm*')

== system proyecto/Modelo NL con Tmod y PID ==
  note: CONSIGNA VELOCIDAD
  note: CONTROLADOR CON TMOD Y PID
  note: SISTEMA FÍSICO
  Corrientes abc : Scope  NumInputPorts=3
  Corrientes qd0 : Scope  NumInputPorts=3
  Gain : Gain  Gain=Pp
  Gain1 : Gain  Gain=1/r
  Gain8 : Gain  Gain=Pp
  Modulador de Tensión : Subsystem
  Modulador de Torque : Subsystem
  PID_vel : Subsystem
  Posición y Velocidad : Scope  NumInputPorts=2
  Resistencia y Temperatura : Scope  NumInputPorts=2
  Sensor de Corriente : Subsystem
  Sensor de posición : Gain
  Sensor de velocidad : Gain
  Tensiones abc : Scope  NumInputPorts=3
  Tensiones qd0 : Scope  NumInputPorts=3
  Tl : Subsystem  Tag=STV Subsys  LoadFcn=sigbuilder_block('load');  StartFcn=sigbuilder_block('start');  StopFcn=sigbuilder_block('stop');  ClipboardFcn=sigbuilder_block('clipboard');  mask(Sigbuilder block){tuvar=[0:10]}
      mask help: Simulink:masks:SigbuilderBlock_MD
      mask init:
      | if ~strcmp(get_param(bdroot(gcbh),'SimulationStatus'),'stopped') tuvar = sigbuilder_block('maskInit'); end
      settings: CopyFcn=sigbuilder_block('copy');  DeleteFcn=sigbuilder_block('delete');  ModelCloseFcn=sigbuilder_block('modelClose');  PreSaveFcn=sigbuilder_block('preSave');  PauseFcn=sigbuilder_block('pause');  ContinueFcn=sigbuilder_block('continue');  NameChangeFcn=sigbuilder_block('namechange');  OpenFcn=sigbuilder_block('open',[5.5 30 1269 678 ]);  CloseFcn=sigbuilder_block('close');
      mask Display: plot(0, 0, 100, 100,[2, 2, 32, 32, 2], [68, 8, 8, 68, 68],[32, 2], [38, 38], [32, 19, 2],[53, 60, 44], [32, 17, 17, 2],[16, 16, 31, 31]);txt = getActiveGroup(gcbh);text(2, 100, txt,'verticalAlignment', 'top');
  inverse_park_transform : MATLAB Function  TreatAsAtomicUnit=on
  inverse_park_transform1 : MATLAB Function  TreatAsAtomicUnit=on
  park_transform : MATLAB Function  TreatAsAtomicUnit=on
  park_transform1 : MATLAB Function  TreatAsAtomicUnit=on
  sub_mecanico_electrico : Subsystem
  sub_termico : Subsystem
  wires:
  Tl/1(Tl) -> Gain1/1
  inverse_park_transform/3(fc) -> Sensor de Corriente/3(In3)
  Sensor de Corriente/3(Out3) -> park_transform1/3(fc), Corrientes abc/3, sub_termico/3(ic)  "Ic*"
  inverse_park_transform/2(fb) -> Sensor de Corriente/2(In2)
  sub_termico/1(Rs) -> Resistencia y Temperatura/1  "Rs"
  Modulador de Tensión/1(Out1) -> park_transform/1(fa)  "Va"
  Sensor de Corriente/1(Out1) -> park_transform1/1(fa), Corrientes abc/1, sub_termico/1(ia)  "Ia*"
  park_transform/1(fq) -> sub_mecanico_electrico/1(Vq)
  sub_mecanico_electrico/1(iq) -> inverse_park_transform/1(fq)
  park_transform1/1(fq) -> Modulador de Torque/2(Iq*), Corrientes qd0/1  "Iq*"
  park_transform/3(f0) -> sub_mecanico_electrico/3(V0)
  park_transform/2(fd) -> sub_mecanico_electrico/2(Vd)
  Gain8/1 -> park_transform1/4(theta_r), inverse_park_transform1/4(theta_r)  "theta_r*"
  park_transform1/2(fd) -> Modulador de Torque/3(Id*), Corrientes qd0/2  "Id*"
  inverse_park_transform/1(fa) -> Sensor de Corriente/1(In1)
  Gain/1 -> inverse_park_transform/4(theta_r), park_transform/4(theta_r)
  sub_mecanico_electrico/5(theta_m) -> Sensor de posición/1, Gain/1
  sub_mecanico_electrico/3(i0) -> inverse_park_transform/3(f0)
  Gain1/1 -> sub_mecanico_electrico/4(T_l_eq)  "Tleq"
  Sensor de velocidad/1 -> PID_vel/2(w_m*), Modulador de Torque/5(w_m*), Posición y Velocidad/2  "w_m*"
  Modulador de Tensión/2(Out2) -> park_transform/2(fb)  "Vb"
  inverse_park_transform1/2(fb) -> Modulador de Tensión/2(fb), Tensiones abc/2  "Vb*"
  inverse_park_transform1/3(fc) -> Modulador de Tensión/3(fc), Tensiones abc/3  "Vc*"
  inverse_park_transform1/1(fa) -> Tensiones abc/1, Modulador de Tensión/1(fa)  "Va*"
  Sensor de posición/1 -> Gain8/1, Posición y Velocidad/1  "theta_m*"
  sub_mecanico_electrico/2(id) -> inverse_park_transform/2(fd)
  Modulador de Tensión/3(Out3) -> park_transform/3(fc)  "Vc"
  sub_mecanico_electrico/4(w_m) -> Sensor de velocidad/1
  Sensor de Corriente/2(Out2) -> park_transform1/2(fb), Corrientes abc/2, sub_termico/2(ib)  "Ib*"
  sub_termico/2(Ts) -> Resistencia y Temperatura/2  "Ts"
  park_transform1/3(f0) -> Modulador de Torque/4(I0*), Corrientes qd0/3  "I0*"
  Modulador de Torque/1(Vq*) -> Tensiones qd0/1, inverse_park_transform1/1(fq)  "Vq*"
  Modulador de Torque/2(Vd*) -> Tensiones qd0/2, inverse_park_transform1/2(fd)  "Vd*"
  Modulador de Torque/3(V0*) -> inverse_park_transform1/3(f0), Tensiones qd0/3  "V0*"
  PID_vel/1(Tm*) -> Modulador de Torque/1(Tm*')
  ? -> PID_vel/1(w_m)

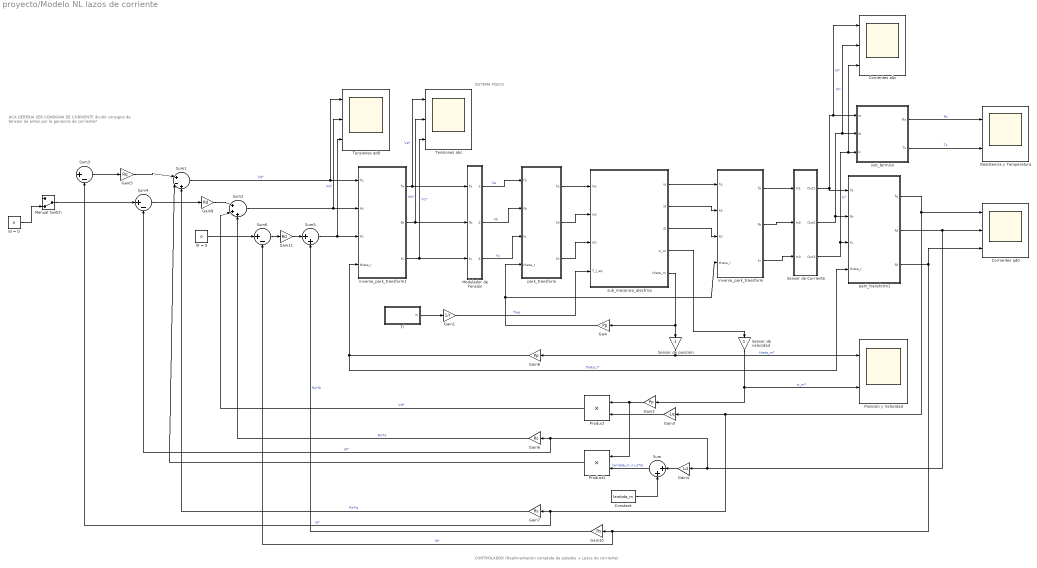
== system proyecto/Modelo NL lazos de corriente ==
  note: ACA DEBERIA SER CONSIGNA DE CORRIENTE
      | dividir consigna de tension de antes por la ganancia de corriente?
  note: CONTROLADOR (Realimentacion completa de estados + Lazos de corriente)
  note: SISTEMA FÍSICO
  Constant : Constant  Value=lambda_m
  Corrientes abc : Scope  NumInputPorts=3
  Corrientes qd0 : Scope  NumInputPorts=3
  Gain : Gain  Gain=Pp
  Gain1 : Gain  Gain=1/r
  Gain10 : Gain  Gain=Rs
  Gain11 : Gain  Gain=R0
  Gain2 : Gain  Gain=Pp
  Gain3 : Gain  Gain=-Lq
  Gain4 : Gain  Gain=Ld
  Gain5 : Gain  Gain=Rq
  Gain6 : Gain  Gain=Rs
  Gain7 : Gain  Gain=Rs
  Gain8 : Gain  Gain=Pp
  Gain9 : Gain  Gain=Rd
  I0 = 0 : Constant  Value=0
  Id = 0 : Constant  Value=0
  Manual Switch : ManualSwitch  CurrentSetting=0
  Modulador de Tensión : Subsystem
  Posición y Velocidad : Scope  NumInputPorts=2
  Product : Product
  Product1 : Product
  Resistencia y Temperatura : Scope  NumInputPorts=2
  Sensor de Corriente : Subsystem
  Sensor de posición : Gain
  Sensor de velocidad : Gain
  Sum : Sum  Inputs=|++
  Sum1 : Sum  Inputs=|+-+
  Sum2 : Sum  Inputs=|+++
  Sum3 : Sum  Inputs=|+-
  Sum4 : Sum  Inputs=|+-
  Sum5 : Sum  Inputs=|++
  Sum6 : Sum  Inputs=|+-
  Tensiones abc : Scope  NumInputPorts=3
  Tensiones qd0 : Scope  NumInputPorts=3
  Tl : Subsystem  Tag=STV Subsys  LoadFcn=sigbuilder_block('load');  StartFcn=sigbuilder_block('start');  StopFcn=sigbuilder_block('stop');  ClipboardFcn=sigbuilder_block('clipboard');  mask(Sigbuilder block){tuvar=[0:10]}
      mask help: Simulink:masks:SigbuilderBlock_MD
      mask init:
      | if ~strcmp(get_param(bdroot(gcbh),'SimulationStatus'),'stopped') tuvar = sigbuilder_block('maskInit'); end
      settings: CopyFcn=sigbuilder_block('copy');  DeleteFcn=sigbuilder_block('delete');  ModelCloseFcn=sigbuilder_block('modelClose');  PreSaveFcn=sigbuilder_block('preSave');  PauseFcn=sigbuilder_block('pause');  ContinueFcn=sigbuilder_block('continue');  NameChangeFcn=sigbuilder_block('namechange');  OpenFcn=sigbuilder_block('open',[5.5 30 1269 678 ]);  CloseFcn=sigbuilder_block('close');
      mask Display: plot(0, 0, 100, 100,[2, 2, 32, 32, 2], [68, 8, 8, 68, 68],[32, 2], [38, 38], [32, 19, 2],[53, 60, 44], [32, 17, 17, 2],[16, 16, 31, 31]);txt = getActiveGroup(gcbh);text(2, 100, txt,'verticalAlignment', 'top');
  inverse_park_transform : MATLAB Function  TreatAsAtomicUnit=on
  inverse_park_transform1 : MATLAB Function  TreatAsAtomicUnit=on
  park_transform : MATLAB Function  TreatAsAtomicUnit=on
  park_transform1 : MATLAB Function  TreatAsAtomicUnit=on
  sub_mecanico_electrico : Subsystem
  sub_termico : Subsystem
  wires:
  Sum4/1 -> Gain9/1
  Tl/1(Tl) -> Gain1/1
  inverse_park_transform/3(fc) -> Sensor de Corriente/3(In3)
  Sensor de Corriente/3(Out3) -> park_transform1/3(fc), Corrientes abc/3, sub_termico/3(ic)  "Ic*"
  Gain3/1 -> Product/2
  park_transform1/3(f0) -> Sum6/2, Gain10/1, Corrientes qd0/3  "I0*"
  Product1/1 -> Sum1/2
  inverse_park_transform/2(fb) -> Sensor de Corriente/2(In2)
  sub_termico/1(Rs) -> Resistencia y Temperatura/1  "Rs"
  Modulador de Tensión/1(Out1) -> park_transform/1(fa)  "Va"
  Sensor de Corriente/1(Out1) -> park_transform1/1(fa), Corrientes abc/1, sub_termico/1(ia)  "Ia*"
  park_transform/1(fq) -> sub_mecanico_electrico/1(Vq)
  sub_mecanico_electrico/1(iq) -> inverse_park_transform/1(fq)
  Sum1/1 -> Tensiones qd0/1, inverse_park_transform1/1(fq)  "Vq*"
  park_transform1/1(fq) -> Sum3/2, Gain7/1, Gain3/1, Corrientes qd0/1  "Iq*"
  park_transform/3(f0) -> sub_mecanico_electrico/3(V0)
  park_transform/2(fd) -> sub_mecanico_electrico/2(Vd)
  Gain8/1 -> park_transform1/4(theta_r), inverse_park_transform1/4(theta_r)  "theta_r*"
  park_transform1/2(fd) -> Sum4/2, Gain6/1, Gain4/1, Corrientes qd0/2  "Id*"
  inverse_park_transform/1(fa) -> Sensor de Corriente/1(In1)
  Gain4/1 -> Sum/1
  Gain/1 -> inverse_park_transform/4(theta_r), park_transform/4(theta_r)
  sub_mecanico_electrico/5(theta_m) -> Sensor de posición/1, Gain/1
  Constant/1 -> Sum/2
  sub_mecanico_electrico/3(i0) -> inverse_park_transform/3(f0)
  Gain1/1 -> sub_mecanico_electrico/4(T_l_eq)  "Tleq"
  Gain2/1 -> Product1/1, Product/1
  Sensor de velocidad/1 -> Gain2/1, Posición y Velocidad/2  "w_m*"
  Sum/1 -> Product1/2  "lambda_m + Ld*Id"
  Modulador de Tensión/2(Out2) -> park_transform/2(fb)  "Vb"
  inverse_park_transform1/2(fb) -> Modulador de Tensión/2(fb), Tensiones abc/2  "Vb*"
  inverse_park_transform1/3(fc) -> Modulador de Tensión/3(fc), Tensiones abc/3  "Vc*"
  inverse_park_transform1/1(fa) -> Tensiones abc/1, Modulador de Tensión/1(fa)  "Va*"
  Sensor de posición/1 -> Gain8/1, Posición y Velocidad/1  "theta_m*"
  sub_mecanico_electrico/2(id) -> inverse_park_transform/2(fd)
  Modulador de Tensión/3(Out3) -> park_transform/3(fc)  "Vc"
  Gain6/1 -> Sum2/3  "Rs*Id"
  Sum2/1 -> Tensiones qd0/2, inverse_park_transform1/2(fd)  "Vd*"
  sub_mecanico_electrico/4(w_m) -> Sensor de velocidad/1
  Product/1 -> Sum2/2  "Vd*"
  Sensor de Corriente/2(Out2) -> park_transform1/2(fb), Corrientes abc/2, sub_termico/2(ib)  "Ib*"
  sub_termico/2(Ts) -> Resistencia y Temperatura/2  "Ts"
  Gain7/1 -> Sum1/3  "Rs*Iq"
  Sum3/1 -> Gain5/1
  Gain5/1 -> Sum1/1
  Gain9/1 -> Sum2/1
  Manual Switch/1 -> Sum4/1
  ? -> Sum3/1
  Id = 0/1 -> Manual Switch/2
  ? -> Manual Switch/1
  Gain11/1 -> Sum5/1
  Sum5/1 -> Tensiones qd0/3, inverse_park_transform1/3(f0)
  Gain10/1 -> Sum5/2  "Rs*I0"
  Sum6/1 -> Gain11/1
  I0 = 0/1 -> Sum6/1

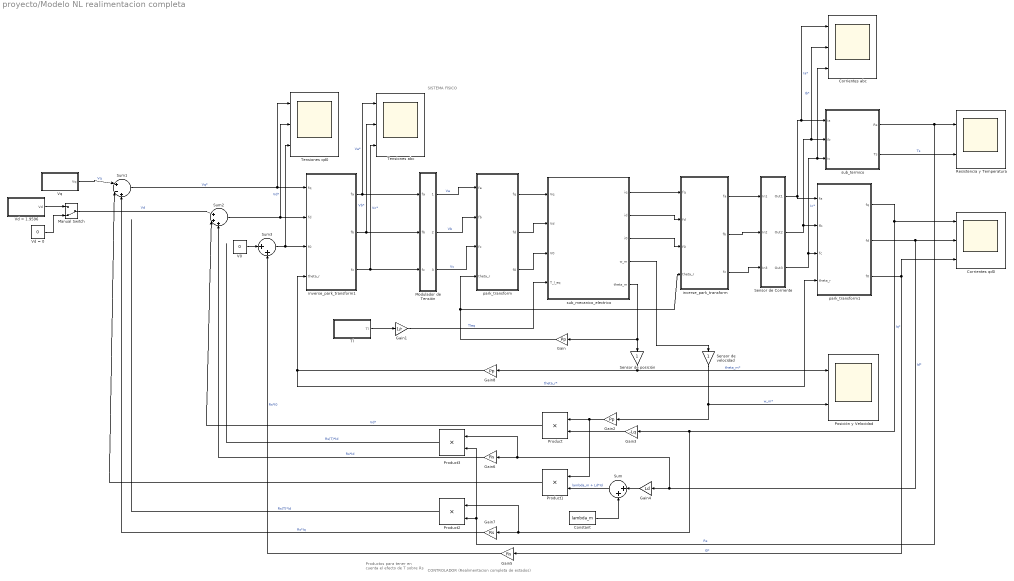
== system proyecto/Modelo NL realimentacion completa ==
  note: Productos para tener en cuenta el efecto de T sobre Rs
  note: CONTROLADOR (Realimentacion completa de estados)
  note: SISTEMA FÍSICO
  Constant : Constant  Value=lambda_m
  Corrientes abc : Scope  NumInputPorts=3
  Corrientes qd0 : Scope  NumInputPorts=3
  Gain : Gain  Gain=Pp
  Gain1 : Gain  Gain=1/r
  Gain2 : Gain  Gain=Pp
  Gain3 : Gain  Gain=-Lq
  Gain4 : Gain  Gain=Ld
  Gain5 : Gain  Gain=Rs
  Gain6 : Gain  Gain=Rs
  Gain7 : Gain  Gain=Rs
  Gain8 : Gain  Gain=Pp
  Manual Switch : ManualSwitch  CurrentSetting=0
  Modulador de Tensión : Subsystem
  Posición y Velocidad : Scope  NumInputPorts=2
  Product{,1..3} (4 alike) : Product
  Resistencia y Temperatura : Scope  NumInputPorts=2
  Sensor de Corriente : Subsystem
  Sensor de posición : Gain
  Sensor de velocidad : Gain
  Sum : Sum  Inputs=|++
  Sum1 : Sum  Inputs=|+-+
  Sum2 : Sum  Inputs=|+++
  Sum3 : Sum  Inputs=|++
  Tensiones abc : Scope  NumInputPorts=3
  Tensiones qd0 : Scope  NumInputPorts=3
  Tl : Subsystem  Tag=STV Subsys  LoadFcn=sigbuilder_block('load');  StartFcn=sigbuilder_block('start');  StopFcn=sigbuilder_block('stop');  ClipboardFcn=sigbuilder_block('clipboard');  mask(Sigbuilder block){tuvar=[0:10]}
      mask help: Simulink:masks:SigbuilderBlock_MD
      mask init:
      | if ~strcmp(get_param(bdroot(gcbh),'SimulationStatus'),'stopped') tuvar = sigbuilder_block('maskInit'); end
      settings: CopyFcn=sigbuilder_block('copy');  DeleteFcn=sigbuilder_block('delete');  ModelCloseFcn=sigbuilder_block('modelClose');  PreSaveFcn=sigbuilder_block('preSave');  PauseFcn=sigbuilder_block('pause');  ContinueFcn=sigbuilder_block('continue');  NameChangeFcn=sigbuilder_block('namechange');  OpenFcn=sigbuilder_block('open',[5.5 30 1269 678 ]);  CloseFcn=sigbuilder_block('close');
      mask Display: plot(0, 0, 100, 100,[2, 2, 32, 32, 2], [68, 8, 8, 68, 68],[32, 2], [38, 38], [32, 19, 2],[53, 60, 44], [32, 17, 17, 2],[16, 16, 31, 31]);txt = getActiveGroup(gcbh);text(2, 100, txt,'verticalAlignment', 'top');
  V0 : Constant  Value=0
  Vd = 0 : Constant  Value=0
  Vd = 1.9596 : Subsystem  Tag=STV Subsys  LoadFcn=sigbuilder_block('load');  StartFcn=sigbuilder_block('start');  StopFcn=sigbuilder_block('stop');  ClipboardFcn=sigbuilder_block('clipboard');  mask(Sigbuilder block){tuvar=[0:10]}
      mask help: Simulink:masks:SigbuilderBlock_MD
      mask init:
      | if ~strcmp(get_param(bdroot(gcbh),'SimulationStatus'),'stopped') tuvar = sigbuilder_block('maskInit'); end
      settings: CopyFcn=sigbuilder_block('copy');  DeleteFcn=sigbuilder_block('delete');  ModelCloseFcn=sigbuilder_block('modelClose');  PreSaveFcn=sigbuilder_block('preSave');  PauseFcn=sigbuilder_block('pause');  ContinueFcn=sigbuilder_block('continue');  NameChangeFcn=sigbuilder_block('namechange');  OpenFcn=sigbuilder_block('open',[5.5 30 1269 678 ]);  CloseFcn=sigbuilder_block('close');
      mask Display: plot(0, 0, 100, 100,[2, 2, 32, 32, 2], [68, 8, 8, 68, 68],[32, 2], [38, 38], [32, 19, 2],[53, 60, 44], [32, 17, 17, 2],[16, 16, 31, 31]);txt = getActiveGroup(gcbh);text(2, 100, txt,'verticalAlignment', 'top');
  Vq : Subsystem  Tag=STV Subsys  LoadFcn=sigbuilder_block('load');  StartFcn=sigbuilder_block('start');  StopFcn=sigbuilder_block('stop');  ClipboardFcn=sigbuilder_block('clipboard');  mask(Sigbuilder block){tuvar=[0:10]}
      mask help: Simulink:masks:SigbuilderBlock_MD
      mask init:
      | if ~strcmp(get_param(bdroot(gcbh),'SimulationStatus'),'stopped') tuvar = sigbuilder_block('maskInit'); end
      settings: CopyFcn=sigbuilder_block('copy');  DeleteFcn=sigbuilder_block('delete');  ModelCloseFcn=sigbuilder_block('modelClose');  PreSaveFcn=sigbuilder_block('preSave');  PauseFcn=sigbuilder_block('pause');  ContinueFcn=sigbuilder_block('continue');  NameChangeFcn=sigbuilder_block('namechange');  OpenFcn=sigbuilder_block('open',[5.5 30 1269 678 ]);  CloseFcn=sigbuilder_block('close');
      mask Display: plot(0, 0, 100, 100,[2, 2, 32, 32, 2], [68, 8, 8, 68, 68],[32, 2], [38, 38], [32, 19, 2],[53, 60, 44], [32, 17, 17, 2],[16, 16, 31, 31]);txt = getActiveGroup(gcbh);text(2, 100, txt,'verticalAlignment', 'top');
  inverse_park_transform : MATLAB Function  TreatAsAtomicUnit=on
  inverse_park_transform1 : MATLAB Function  TreatAsAtomicUnit=on
  park_transform : MATLAB Function  TreatAsAtomicUnit=on
  park_transform1 : MATLAB Function  TreatAsAtomicUnit=on
  sub_mecanico_electrico : Subsystem
  sub_termico : Subsystem
  wires:
  sub_mecanico_electrico/2(id) -> inverse_park_transform/2(fd)
  Sensor de posición/1 -> Gain8/1, Posición y Velocidad/1  "theta_m*"
  inverse_park_transform1/3(fc) -> Modulador de Tensión/3(fc), Tensiones abc/3  "Vc*"
  Vq/1(Vq) -> Sum1/1  "Vq"
  inverse_park_transform1/2(fb) -> Modulador de Tensión/2(fb), Tensiones abc/2  "Vb*"
  sub_termico/2(Ts) -> Resistencia y Temperatura/2  "Ts"
  Gain2/1 -> Product1/1, Product/1
  sub_mecanico_electrico/3(i0) -> inverse_park_transform/3(f0)
  Gain1/1 -> sub_mecanico_electrico/4(T_l_eq)  "Tleq"
  sub_mecanico_electrico/5(theta_m) -> Sensor de posición/1, Gain/1
  Gain4/1 -> Sum/1
  inverse_park_transform/1(fa) -> Sensor de Corriente/1(In1)
  Sum/1 -> Product1/2  "lambda_m + Ld*Id"
  Gain/1 -> inverse_park_transform/4(theta_r), park_transform/4(theta_r)
  Modulador de Tensión/2(Out2) -> park_transform/2(fb)  "Vb"
  Gain3/1 -> Product/2
  Product/1 -> Sum2/2  "Vd*"
  Sensor de Corriente/3(Out3) -> park_transform1/3(fc), Corrientes abc/3, sub_termico/3(ic)  "Ic*"
  inverse_park_transform/3(fc) -> Sensor de Corriente/3(In3)
  Manual Switch/1 -> Sum2/1  "Vd"
  Tl/1(Tl) -> Gain1/1
  Sensor de Corriente/2(Out2) -> park_transform1/2(fb), Corrientes abc/2, sub_termico/2(ib)  "Ib*"
  inverse_park_transform1/1(fa) -> Tensiones abc/1, Modulador de Tensión/1(fa)  "Va*"
  park_transform/2(fd) -> sub_mecanico_electrico/2(Vd)
  Modulador de Tensión/3(Out3) -> park_transform/3(fc)  "Vc"
  sub_mecanico_electrico/4(w_m) -> Sensor de velocidad/1
  Sensor de velocidad/1 -> Gain2/1, Posición y Velocidad/2  "w_m*"
  park_transform/3(f0) -> sub_mecanico_electrico/3(V0)
  Gain8/1 -> park_transform1/4(theta_r), inverse_park_transform1/4(theta_r)  "theta_r*"
  Sum2/1 -> Tensiones qd0/2, inverse_park_transform1/2(fd)  "Vd*"
  park_transform1/1(fq) -> Product2/1, Gain7/1, Gain3/1, Corrientes qd0/1  "Iq*"
  Constant/1 -> Sum/2
  Sum1/1 -> Tensiones qd0/1, inverse_park_transform1/1(fq)  "Vq*"
  park_transform/1(fq) -> sub_mecanico_electrico/1(Vq)
  sub_mecanico_electrico/1(iq) -> inverse_park_transform/1(fq)
  Sensor de Corriente/1(Out1) -> park_transform1/1(fa), Corrientes abc/1, sub_termico/1(ia)  "Ia*"
  Product1/1 -> Sum1/2
  Modulador de Tensión/1(Out1) -> park_transform/1(fa)  "Va"
  inverse_park_transform/2(fb) -> Sensor de Corriente/2(In2)
  sub_termico/1(Rs) -> Product2/2, Product3/2, Resistencia y Temperatura/1  "Rs"
  park_transform1/2(fd) -> Product3/1, Gain6/1, Gain4/1, Corrientes qd0/2  "Id*"
  park_transform1/3(f0) -> Gain5/1, Corrientes qd0/3  "I0*"
  Gain6/1 -> Sum2/3  "Rs*Id"
  Gain7/1 -> Sum1/3  "Rs*Iq"
  Product2/1 -> ?  "Rs(T)*Id"
  Product3/1 -> ?  "Rs(T)*Id"
  Vd = 1.9596/1(Vd) -> Manual Switch/1
  Vd = 0/1 -> Manual Switch/2
  V0/1 -> Sum3/1
  Sum3/1 -> Tensiones qd0/3, inverse_park_transform1/3(f0)
  Gain5/1 -> Sum3/2  "Rs*I0"

== system proyecto/Modelo NL virtual ==
  Va : Inport
  Vb : Inport  Port=2
  Vc : Inport  Port=3
  Tl : Inport  Port=4
  Gain : Gain  Gain=Pp
  Gain1 : Gain  Gain=1/r
  inverse_park_transform : MATLAB Function  TreatAsAtomicUnit=on
  park_transform : MATLAB Function  TreatAsAtomicUnit=on
  sub_mecanico_electrico : Subsystem
  sub_termico : Subsystem
  theta_m : Outport
  w_m : Outport  Port=2
  ia : Outport  Port=3
  ib : Outport  Port=4
  ic : Outport  Port=5
  Rs : Outport  Port=6
  Ts : Outport  Port=7
  wires:
  Gain/1 -> inverse_park_transform/4(theta_r), park_transform/4(theta_r)
  Tl/1 -> Gain1/1
  Gain1/1 -> sub_mecanico_electrico/4(V0)
  park_transform/1(fq) -> sub_mecanico_electrico/1(T_l_eq)
  park_transform/2(fd) -> sub_mecanico_electrico/2(Vq)
  park_transform/3(f0) -> sub_mecanico_electrico/3(Vd)
  Va/1 -> park_transform/1(fa)
  Vb/1 -> park_transform/2(fb)
  Vc/1 -> park_transform/3(fc)
  inverse_park_transform/1(fa) -> sub_termico/1(ia), ia/1
  inverse_park_transform/2(fb) -> sub_termico/2(ib), ib/1
  inverse_park_transform/3(fc) -> sub_termico/3(ic), ic/1
  sub_termico/1(Rs) -> Rs/1
  sub_termico/2(Ts) -> Ts/1
  sub_mecanico_electrico/5(theta_m) -> theta_m/1, Gain/1
  sub_mecanico_electrico/1(w_m) -> w_m/1
  sub_mecanico_electrico/2(iq) -> inverse_park_transform/1(fq)
  sub_mecanico_electrico/3(id) -> inverse_park_transform/2(fd)
  sub_mecanico_electrico/4(i0) -> inverse_park_transform/3(f0)

== system proyecto/Modulador de Torque ==
  Iq* : Inport
  Id* : Inport  Port=2
  I0* : Inport  Port=3
  w_m* : Inport  Port=4
  Tm*' : Inport  Port=5
  Constant1 : Constant  Value=lambda_m
  "Ecuacion Tm 3.5, Id = 0" : Gain  Gain=1/(3/2*Pp*lambda_m)
  "Ecuacion Tm 3.5, estrategia general" : Subsystem
  Gain1 : Gain  Gain=Pp
  Gain10 : Gain  Gain=b_eq
  Gain11 : Gain  Gain=R0
  Gain13 : Gain  Gain=Ld
  Gain14 : Gain  Gain=Rs
  Gain15 : Gain  Gain=Rs
  Gain16 : Gain  Gain=Rs
  Gain5 : Gain  Gain=Rq
  Gain8 : Gain  Gain=-Lq
  Gain9 : Gain  Gain=Rd
  I0 = 0 : Constant  Value=0
  Id : Constant  Value=0
  Product2 : Product
  Product3 : Product
  Sum1 : Sum  Inputs=|+-+
  Sum2 : Sum  Inputs=|+++
  Sum3 : Sum  Inputs=|+-
  Sum4 : Sum  Inputs=|+-
  Sum5 : Sum  Inputs=|++
  Sum6 : Sum  Inputs=|++
  Sum7 : Sum  Inputs=|+-
  Sum8 : Sum  Inputs=|++
  Vq* : Outport
  Vd* : Outport  Port=2
  V0* : Outport  Port=3
  wires:
  Sum7/1 -> Gain11/1
  I0 = 0/1 -> Sum7/1
  "Ecuacion Tm 3.5, estrategia general"/1(Iq*') -> ?  "Iq*'"
  Tm*'/1 -> Sum5/1
  "Ecuacion Tm 3.5, Id = 0"/1 -> Sum3/1  "Iq*"
  Sum4/1 -> Gain9/1
  Sum5/1 -> "Ecuacion Tm 3.5, Id = 0"/1, "Ecuacion Tm 3.5, estrategia general"/1(Tm*')
  Id/1 -> Sum4/1
  Gain5/1 -> Sum1/1
  Gain9/1 -> Sum2/1
  Sum3/1 -> Gain5/1
  Sum2/1 -> Vd*/1  "Vd*"
  Gain11/1 -> Sum6/1
  Sum1/1 -> Vq*/1  "Vq*"
  Gain10/1 -> Sum5/2  "b_eq * w_m*"
  Gain14/1 -> Sum1/3  "Rs*Iq"
  Product2/1 -> Sum2/2  "-Pp*w_m*Lq*Iq"
  Gain15/1 -> Sum2/3  "Rs*Id"
  Gain16/1 -> Sum6/2  "Rs*I0"
  Product3/1 -> Sum1/2  "Pp*w_m*(lambda_m+Ld*Id)"
  w_m*/1 -> Gain10/1, Gain1/1  "w_m*"
  Iq*/1 -> Sum3/2, Gain14/1, Gain8/1  "Iq*"
  Gain13/1 -> Sum8/1
  Gain8/1 -> Product2/2
  Gain1/1 -> Product3/1, Product2/1
  Constant1/1 -> Sum8/2
  Sum8/1 -> Product3/2  "lambda_m + Ld*Id"
  Id*/1 -> "Ecuacion Tm 3.5, estrategia general"/2(Id*), Sum4/2, Gain15/1, Gain13/1  "Id*"
  I0*/1 -> Sum7/2, Gain16/1  "I0*"
  Sum6/1 -> V0*/1  "V0*"

== system proyecto/Observador ==
  theta_m : Inport
  Tm** : Inport  Port=2
  Gain : Gain  Gain=1/Jeq
  Gain1 : Gain  Gain=Kw
  Gain2 : Gain  Gain=Ktheta
  Integrator : Integrator
  Integrator1 : Integrator
  Sum : Sum  Inputs=+|-
  Sum1 : Sum  Inputs=++|
  Sum2 : Sum  Inputs=++|
  theta_obs : Outport
  w_obs1 : Outport  Port=2
  w_obs2 : Outport  Port=3
  wires:
  Integrator/1 -> Sum/2, theta_obs/1
  Sum1/1 -> w_obs1/1, Integrator/1
  Sum2/1 -> w_obs2/1, Integrator1/1
  Sum/1 -> Gain2/1, Gain1/1
  theta_m/1 -> Sum/1
  Tm**/1 -> Gain/1
  Gain/1 -> Sum2/2
  Gain1/1 -> Sum2/1
  Gain2/1 -> Sum1/1
  Integrator1/1 -> Sum1/2
